simulink model "snap2_f_200msps_64i_4096c_test"  (R2019a)
settings: Solver=VariableStepDiscrete  StartTime=0.0  StopTime=10.0  RelTol=1e-3
libraries: xbsIndex_r4 x8040, casper_library_misc x13, xps_library x6, casper_library_delays x4, casper_library_sources x4, casper_library_reorder x2
(part 11 of 84)

== system snap2_f_200msps_64i_4096c_test/input/bit_stats ==
  din : Inport
  Counter1 : xbsIndex_r4/Counter  cnt_type=Free Running  cnt_to=Inf  operation=Up  start_count=0  cnt_by_val=1  arith_type=Unsigned  n_bits=20  bin_pt=0  load_pin=off  rst=off  en=off  explicit_period=on  period=1  use_behavioral_HDL=off  implementation=Fabric  use_rpm=on  dbl_ovrd=off  block_type=counter
      settings: xl_area=[0, 0, 0, 0, 0, 0, 0]
  Mux : xbsIndex_r4/Mux  inputs=32  en=off  latency=1  precision=Full  arith_type=Unsigned  n_bits=16  bin_pt=14  quantization=Truncate  overflow=Wrap  dbl_ovrd=off  block_type=mux
  Mux1 : xbsIndex_r4/Mux  inputs=2  en=off  latency=1  precision=Full  arith_type=Unsigned  n_bits=16  bin_pt=14  quantization=Truncate  overflow=Wrap  dbl_ovrd=off  block_type=mux
  Slice1 : xbsIndex_r4/Slice  nbits=1  boolean_output=on  mode=Upper Bit Location + Width  bit1=0  base1=MSB of Input  bit0=19  base0=LSB of Input  dbl_ovrd=off  block_type=slice
      settings: infoedit="Extracts a given range of bits from each input sample and presents it at the output.  The output type is ordinarily unsigned with binary point at zero, but can be Boolean when the slice is one bit wide.<P><P>Hardware notes: In hardware this block costs nothing."  block_version=10.1.3
  Slice2 : xbsIndex_r4/Slice  nbits=1  boolean_output=off  mode=Lower Bit Location + Width  bit1=0  base1=MSB of Input  bit0=5  base0=LSB of Input  dbl_ovrd=off  block_type=slice
      settings: block_version=10.1.3
  Slice3 : xbsIndex_r4/Slice  nbits=5  boolean_output=off  mode=Lower Bit Location + Width  bit1=0  base1=MSB of Input  bit0=0  base0=LSB of Input  dbl_ovrd=off  block_type=slice
      settings: block_version=10.1.3
  bus_expand1 : Subsystem  AncestorBlock=casper_library_flow_control/bus_expand  mask(bus_expand){mode=divisions of equal size, outputNum=32, outputWidth=10, outputBinaryPt=0, outputArithmeticType=0, show_format=off, outputToWorkspace=off, variablePrefix=out, outputToModelAsWell=on}
      mask prompts: outputNum "Number of outputs:"; outputWidth "Output width:"; outputBinaryPt "Output binary point position:"; outputArithmeticType "Output arithmetic type (ufix=0, fix=1, bool=2):"; show_format "Print format string?"; outputToWorkspace "Output to workspace?"; variablePrefix "Variable name prefix:"; outputToModelAsWell "Output to model as well?"
      mask help:
      | Expands a 'bus' made using a bus_create or Xilinx
      | concat block.
      | The input will be divided into the specified number
      | of outputs with the specified arithmetic types.
      | Divisions are made from most significant bit.
      mask init: same as snap2_f_200msps_64i_4096c_test/chan_reorder/bus_expand2
      settings: AttributesFormatString=32 outputs
      mask TypeOptions mode: divisions of equal size | divisions of arbitrary size
      mask Callback mode: bus_expand_callback();
      mask Callback outputWidth: bus_expand_callback();
      mask Callback outputToWorkspace: bus_expand_callback();
  bus_expand2 : Subsystem  AncestorBlock=casper_library_flow_control/bus_expand  mask(bus_expand){mode=divisions of equal size, outputNum=2, outputWidth=10*32, outputBinaryPt=0, outputArithmeticType=0, show_format=off, outputToWorkspace=off, variablePrefix=out, outputToModelAsWell=on}
      mask prompts: outputNum "Number of outputs:"; outputWidth "Output width:"; outputBinaryPt "Output binary point position:"; outputArithmeticType "Output arithmetic type (ufix=0, fix=1, bool=2):"; show_format "Print format string?"; outputToWorkspace "Output to workspace?"; variablePrefix "Variable name prefix:"; outputToModelAsWell "Output to model as well?"
      mask help:
      | Expands a 'bus' made using a bus_create or Xilinx
      | concat block.
      | The input will be divided into the specified number
      | of outputs with the specified arithmetic types.
      | Divisions are made from most significant bit.
      mask init: same as snap2_f_200msps_64i_4096c_test/chan_reorder/bus_expand2
      settings: AttributesFormatString=2 outputs
      mask TypeOptions mode: divisions of equal size | divisions of arbitrary size
      mask Callback mode: bus_expand_callback();
      mask Callback outputWidth: bus_expand_callback();
      mask Callback outputToWorkspace: bus_expand_callback();
  edge_detect1 : Subsystem  AncestorBlock=casper_library_misc/edge_detect  mask(edge_detect){edge=Rising, polarity=Active High, x_in=[0 0.08 0.08 0.16 0.16 0.24 0.24 0.32 0.32 0.4], y_in=[-1 -1  1  1  1  1  1  1  1  1], x_out=[0.6 0.68 0.68 0.76 0.76 0.84 0.84 0.92 0.92 1], y_out=[-1 -1  1  1 -1 -1 -1 -1 -1 -1]}
      mask prompts: edge "Edge Type"; polarity "Output Polarity"; x_in "Input X Positions"; y_in "Input Y Positions"; x_out "Output X Positions"; y_out "Output Y Positions"
      mask help: Output is active for one-cycle after each edge of the specified type (i.e. rising, falling or both).
      mask init: same as snap2_f_200msps_64i_4096c_test/sync/ed
      settings: AttributesFormatString=|
      | rising edges
      | active high
      mask Help: Output is active for one-cycle after each edge of the specified type (i.e. rising, falling, or both).  Latency is zero.
      mask TypeOptions edge: Rising | Falling | Both
      mask TypeOptions polarity: Active High | Active Low
      mask Display:
      | plot(x_in_num,0.5+y_in_num*0.2);
      | plot(x_out_num,0.5+y_out_num*0.2);
  histogram : Subsystem  mask{bitwidth=10}
  input_sel : Subsystem  Tag=xps:sw_reg  AncestorBlock=xps_library/Memory/software_register  mask(swreg){io_dir=From Processor, io_delay=0, init_val=0, sample_period=1, names=reg, bitwidths=32, bin_pts=0, arith_types=0, sim_port=on, show_format=on}
      mask prompts: io_dir "I/O direction"; io_delay "I/O delay"; init_val "Initial Value"; sample_period "Sample period"; names "Bitfield names [msb...lsb]"; bitwidths "Bitfield widths"; bin_pts "Bitfield binary pts"; arith_types "Bitfield types, ufix=0, fix=1, bool=2"; sim_port "Provide sim input/output?"; show_format "Print format string?"
      mask help: A 32-bit software-accessible register. Can be divided into bitfields of varying widths and types using the fields in the block mask.
      mask init:
      | swreg_init(gcb)
      settings: AttributesFormatString=1input:uf32.0 = 32 bits
      mask TypeOptions io_dir: To Processor | From Processor
      mask Callback io_dir:
      | mask_enables = get_param(gcb, 'MaskEnables');
      | mask_names = get_param(gcb, 'MaskNames');
      | if strcmp(get_param(gcb, 'io_dir'), 'To Processor'),
      |     mask_enables{ismember(mask_names, 'sample_period')} = 'off';
      | else
      |     mask_enables{ismember(mask_names, 'sample_period')} = 'on';
      | end
      | set_param(gcb, 'MaskEnables', mask_enables);
      mask DialogControl ParameterTabVar0 Prompt: Setup
  wires:
  [adc_hist_rst] -> histogram/2(new_acc)
  Mux/1 -> histogram/1(din)
  Counter1/1 -> Slice1/1
  Slice1/1 -> edge_detect1/1(in)
  edge_detect1/1(out) -> [adc_hist_rst]
  input_sel/1(in_reg) -> Slice3/1, Slice2/1
  Slice2/1 -> [sel_msb]
  din/1 -> bus_expand2/1(bus_in)
  bus_expand2/1(msb_out2) -> Mux1/2
  bus_expand2/2(lsb_out1) -> Mux1/3
  Slice3/1 -> [sel_lsb]
  [sel_msb] -> Mux1/1
  Mux1/1 -> bus_expand1/1(bus_in)
  [sel_lsb] -> Mux/1
  bus_expand1/14(out19) -> Mux/15
  bus_expand1/7(out26) -> Mux/8
  bus_expand1/13(out20) -> Mux/14
  bus_expand1/17(out16) -> Mux/18
  bus_expand1/18(out15) -> Mux/19
  bus_expand1/11(out22) -> Mux/12
  bus_expand1/20(out13) -> Mux/21
  bus_expand1/2(out31) -> Mux/3
  bus_expand1/9(out24) -> Mux/10
  bus_expand1/3(out30) -> Mux/4
  bus_expand1/6(out27) -> Mux/7
  bus_expand1/10(out23) -> Mux/11
  bus_expand1/21(out12) -> Mux/22
  bus_expand1/16(out17) -> Mux/17
  bus_expand1/19(out14) -> Mux/20
  bus_expand1/12(out21) -> Mux/13
  bus_expand1/4(out29) -> Mux/5
  bus_expand1/1(msb_out32) -> Mux/2
  bus_expand1/15(out18) -> Mux/16
  bus_expand1/5(out28) -> Mux/6
  bus_expand1/22(out11) -> Mux/23
  bus_expand1/23(out10) -> Mux/24
  bus_expand1/24(out9) -> Mux/25
  bus_expand1/25(out8) -> Mux/26
  bus_expand1/26(out7) -> Mux/27
  bus_expand1/27(out6) -> Mux/28
  bus_expand1/28(out5) -> Mux/29
  bus_expand1/29(out4) -> Mux/30
  bus_expand1/30(out3) -> Mux/31
  bus_expand1/31(out2) -> Mux/32
  bus_expand1/32(lsb_out1) -> Mux/33
  bus_expand1/8(out25) -> Mux/9

== system snap2_f_200msps_64i_4096c_test/input/bus_create2 ==
  in1 : Inport
  in2 : Inport  Port=2
  in3 : Inport  Port=3
  in4 : Inport  Port=4
  concatenate : xbsIndex_r4/Concat  num_inputs=4  dbl_ovrd=off  block_type=concat
  reinterpret{1..4} (4 alike) : xbsIndex_r4/Reinterpret  force_arith_type=on  arith_type=Unsigned  force_bin_pt=on  bin_pt=0  block_type=reinterpret
      reinterpret1 settings: infoedit="Changes signal type without altering the binary representation.   You can changed the signal between signed and unsigned, and relocate the binary point.<br><br>Hardware notes: In hardware this block costs nothing.<br><br>Example:  Suppose the input is 6 bits wide, signed, with 2 fractional bits, and the output is forced to unsigned with 0 fractional bits.  Then an input of -2.0 (1110.00 in binary 2's complement) becomes an output of 56 (111000 in binary)."
      reinterpret2 settings: infoedit="Changes signal type without altering the binary representation.   You can changed the signal between signed and unsigned, and relocate the binary point.<br><br>Hardware notes: In hardware this block costs nothing.<br><br>Example:  Suppose the input is 6 bits wide, signed, with 2 fractional bits, and the output is forced to unsigned with 0 fractional bits.  Then an input of -2.0 (1110.00 in binary 2's complement) becomes an output of 56 (111000 in binary)."
  bus_out : Outport
  wires:
  concatenate/1 -> bus_out/1
  in1/1 -> reinterpret1/1
  reinterpret1/1 -> concatenate/1
  in2/1 -> reinterpret2/1
  reinterpret2/1 -> concatenate/2
  in3/1 -> reinterpret3/1
  reinterpret3/1 -> concatenate/3
  in4/1 -> reinterpret4/1
  reinterpret4/1 -> concatenate/4

== system snap2_f_200msps_64i_4096c_test/input/bus_mux ==
  sel : Inport
  d0 : Inport  Port=2
  d1 : Inport  Port=3
  d2 : Inport  Port=4
  misci : Inport  Port=5
  d_bussify : Subsystem  AncestorBlock=casper_library_flow_control/bus_create  mask(bus_create){inputNum=64}
      mask prompts: inputNum "Number of inputs:"
      mask init:
      | bus_create_init(gcb,...
      |     'inputNum', inputNum);
  dmisc : xbsIndex_r4/Delay  rst=off  infoeditControl=Selection of Reset will increase slice count due to use of real FFs and instead of SRLs  en=off  latency=1  reg_retiming=on  dbl_ovrd=off  block_type=delay
  expand0 : Subsystem  AncestorBlock=casper_library_flow_control/bus_expand  mask(bus_expand){mode=divisions of arbitrary size, outputNum=1, outputWidth=[10;10;10;10;10;10;10;10;10;10;10;10;10;10;10;10;10;10;10;10;10;10;10;10;10;10;10;10;10;10;10;10;10;10;10;10;10;10;10;10;10;10;10;10;10;10;10;10;10;10;10;10;10;10;10;10;10;10;10;10;10;10;10;10], outputBinaryPt=[0  0  0  0  0  0  0  0  0  0  0  0  0  0  0  0  0  0  0  0  0  0  0  0  0  0  0  0  0  0  0  0  0  0  0  0  0  0  0  0  0  0  0  0  0  0  0  0  0  0  0  0  0  0  0  0  0  0  0  0  0  0  0  0], outputArithmeticType=[0  0  0  0  0  0  0  0  0  0  0  0  0  0  0  0  0  0  0  0  0  0  0  0  0  0  0  0  0  0  0  0  0  0  0  0  0  0  0  0  0  0  0  0  0  0  0  0  0  0  0  0  0  0  0  0  0  0  0  0  0  0  0  0], show_format=on, outputToWorkspace=off, variablePrefix=, outputToModelAsWell=on}
      mask prompts: outputNum "Number of outputs:"; outputWidth "Output width [msb ... lsb]:"; outputBinaryPt "Output binary point position [msb ... lsb]:"; outputArithmeticType "Output arithmetic type (ufix=0, fix=1, bool=2) [msb ... lsb]:"; show_format "Print format string?"; outputToWorkspace "Output to workspace?"; variablePrefix "Variable name prefix:"; outputToModelAsWell "Output to model as well?"
      mask help:
      | Expands a 'bus' made using a bus_create or Xilinx
      | concat block.
      | The input will be divided into the specified number
      | of outputs with the specified arithmetic types.
      | Divisions are made from most significant bit.
      mask init: same as snap2_f_200msps_64i_4096c_test/chan_reorder/bus_expand2
      settings: AttributesFormatString=64 outputs: uf10.0,uf10.0,uf10.0,uf10.0,uf10.0,uf10.0,uf10.0,uf10.0,uf10.0,uf10.0,uf10.0,uf10.0,uf10.0,uf10.0,uf10.0,uf10.0,uf10.0,uf10.0,uf10.0,uf10.0,uf10.0,uf10.0,uf10.0,uf10.0,uf10.0,uf10.0,uf10.0,uf10.0,uf10.0,uf10.0,uf10.0,uf10.0,uf10.0,uf10.0,uf10.0,uf10.0,uf10.0,uf10.0,uf10.0,uf10.0,uf10.0,uf10.0,uf10.0,uf10.0,uf10.0,uf10.0,uf10.0,uf10.0,uf10.0,uf10.0,uf10.0,uf10.0,uf10.0,uf10.0,uf10.0,uf10.0,uf10.0,uf10.0,uf10.0,uf10.0,uf10.0,uf10.0,uf10.0,uf10.0,
      mask TypeOptions mode: divisions of equal size | divisions of arbitrary size
      mask Callback mode: bus_expand_callback();
      mask Callback outputWidth: bus_expand_callback();
      mask Callback outputToWorkspace: bus_expand_callback();
  expand1 : Subsystem  AncestorBlock=casper_library_flow_control/bus_expand  mask(bus_expand){mode=divisions of arbitrary size, outputNum=1, outputWidth=[10;10;10;10;10;10;10;10;10;10;10;10;10;10;10;10;10;10;10;10;10;10;10;10;10;10;10;10;10;10;10;10;10;10;10;10;10;10;10;10;10;10;10;10;10;10;10;10;10;10;10;10;10;10;10;10;10;10;10;10;10;10;10;10], outputBinaryPt=[0  0  0  0  0  0  0  0  0  0  0  0  0  0  0  0  0  0  0  0  0  0  0  0  0  0  0  0  0  0  0  0  0  0  0  0  0  0  0  0  0  0  0  0  0  0  0  0  0  0  0  0  0  0  0  0  0  0  0  0  0  0  0  0], outputArithmeticType=[0  0  0  0  0  0  0  0  0  0  0  0  0  0  0  0  0  0  0  0  0  0  0  0  0  0  0  0  0  0  0  0  0  0  0  0  0  0  0  0  0  0  0  0  0  0  0  0  0  0  0  0  0  0  0  0  0  0  0  0  0  0  0  0], show_format=on, outputToWorkspace=off, variablePrefix=, outputToModelAsWell=on}
      mask prompts: outputNum "Number of outputs:"; outputWidth "Output width [msb ... lsb]:"; outputBinaryPt "Output binary point position [msb ... lsb]:"; outputArithmeticType "Output arithmetic type (ufix=0, fix=1, bool=2) [msb ... lsb]:"; show_format "Print format string?"; outputToWorkspace "Output to workspace?"; variablePrefix "Variable name prefix:"; outputToModelAsWell "Output to model as well?"
      mask help:
      | Expands a 'bus' made using a bus_create or Xilinx
      | concat block.
      | The input will be divided into the specified number
      | of outputs with the specified arithmetic types.
      | Divisions are made from most significant bit.
      mask init: same as snap2_f_200msps_64i_4096c_test/chan_reorder/bus_expand2
      settings: AttributesFormatString=64 outputs: uf10.0,uf10.0,uf10.0,uf10.0,uf10.0,uf10.0,uf10.0,uf10.0,uf10.0,uf10.0,uf10.0,uf10.0,uf10.0,uf10.0,uf10.0,uf10.0,uf10.0,uf10.0,uf10.0,uf10.0,uf10.0,uf10.0,uf10.0,uf10.0,uf10.0,uf10.0,uf10.0,uf10.0,uf10.0,uf10.0,uf10.0,uf10.0,uf10.0,uf10.0,uf10.0,uf10.0,uf10.0,uf10.0,uf10.0,uf10.0,uf10.0,uf10.0,uf10.0,uf10.0,uf10.0,uf10.0,uf10.0,uf10.0,uf10.0,uf10.0,uf10.0,uf10.0,uf10.0,uf10.0,uf10.0,uf10.0,uf10.0,uf10.0,uf10.0,uf10.0,uf10.0,uf10.0,uf10.0,uf10.0,
      mask TypeOptions mode: divisions of equal size | divisions of arbitrary size
      mask Callback mode: bus_expand_callback();
      mask Callback outputWidth: bus_expand_callback();
      mask Callback outputToWorkspace: bus_expand_callback();
  expand2 : Subsystem  AncestorBlock=casper_library_flow_control/bus_expand  mask(bus_expand){mode=divisions of arbitrary size, outputNum=1, outputWidth=[10;10;10;10;10;10;10;10;10;10;10;10;10;10;10;10;10;10;10;10;10;10;10;10;10;10;10;10;10;10;10;10;10;10;10;10;10;10;10;10;10;10;10;10;10;10;10;10;10;10;10;10;10;10;10;10;10;10;10;10;10;10;10;10], outputBinaryPt=[0  0  0  0  0  0  0  0  0  0  0  0  0  0  0  0  0  0  0  0  0  0  0  0  0  0  0  0  0  0  0  0  0  0  0  0  0  0  0  0  0  0  0  0  0  0  0  0  0  0  0  0  0  0  0  0  0  0  0  0  0  0  0  0], outputArithmeticType=[0  0  0  0  0  0  0  0  0  0  0  0  0  0  0  0  0  0  0  0  0  0  0  0  0  0  0  0  0  0  0  0  0  0  0  0  0  0  0  0  0  0  0  0  0  0  0  0  0  0  0  0  0  0  0  0  0  0  0  0  0  0  0  0], show_format=on, outputToWorkspace=off, variablePrefix=, outputToModelAsWell=on}
      mask prompts: outputNum "Number of outputs:"; outputWidth "Output width [msb ... lsb]:"; outputBinaryPt "Output binary point position [msb ... lsb]:"; outputArithmeticType "Output arithmetic type (ufix=0, fix=1, bool=2) [msb ... lsb]:"; show_format "Print format string?"; outputToWorkspace "Output to workspace?"; variablePrefix "Variable name prefix:"; outputToModelAsWell "Output to model as well?"
      mask help:
      | Expands a 'bus' made using a bus_create or Xilinx
      | concat block.
      | The input will be divided into the specified number
      | of outputs with the specified arithmetic types.
      | Divisions are made from most significant bit.
      mask init: same as snap2_f_200msps_64i_4096c_test/chan_reorder/bus_expand2
      settings: AttributesFormatString=64 outputs: uf10.0,uf10.0,uf10.0,uf10.0,uf10.0,uf10.0,uf10.0,uf10.0,uf10.0,uf10.0,uf10.0,uf10.0,uf10.0,uf10.0,uf10.0,uf10.0,uf10.0,uf10.0,uf10.0,uf10.0,uf10.0,uf10.0,uf10.0,uf10.0,uf10.0,uf10.0,uf10.0,uf10.0,uf10.0,uf10.0,uf10.0,uf10.0,uf10.0,uf10.0,uf10.0,uf10.0,uf10.0,uf10.0,uf10.0,uf10.0,uf10.0,uf10.0,uf10.0,uf10.0,uf10.0,uf10.0,uf10.0,uf10.0,uf10.0,uf10.0,uf10.0,uf10.0,uf10.0,uf10.0,uf10.0,uf10.0,uf10.0,uf10.0,uf10.0,uf10.0,uf10.0,uf10.0,uf10.0,uf10.0,
      mask TypeOptions mode: divisions of equal size | divisions of arbitrary size
      mask Callback mode: bus_expand_callback();
      mask Callback outputWidth: bus_expand_callback();
      mask Callback outputToWorkspace: bus_expand_callback();
  mux{0..63} (64 alike) : xbsIndex_r4/Mux  inputs=3  en=off  latency=1  precision=Full  arith_type=Unsigned  n_bits=16  bin_pt=14  quantization=Truncate  overflow=Wrap  dbl_ovrd=off  block_type=mux
  sel_expand : Subsystem  AncestorBlock=casper_library_flow_control/bus_expand  mask(bus_expand){mode=divisions of equal size, outputNum=64, outputWidth=2, outputBinaryPt=0, outputArithmeticType=0, show_format=on, outputToWorkspace=off, variablePrefix=, outputToModelAsWell=on}
      mask prompts: outputNum "Number of outputs:"; outputWidth "Output width:"; outputBinaryPt "Output binary point position:"; outputArithmeticType "Output arithmetic type (ufix=0, fix=1, bool=2):"; show_format "Print format string?"; outputToWorkspace "Output to workspace?"; variablePrefix "Variable name prefix:"; outputToModelAsWell "Output to model as well?"
      mask help:
      | Expands a 'bus' made using a bus_create or Xilinx
      | concat block.
      | The input will be divided into the specified number
      | of outputs with the specified arithmetic types.
      | Divisions are made from most significant bit.
      mask init: same as snap2_f_200msps_64i_4096c_test/chan_reorder/bus_expand2
      settings: AttributesFormatString=64 outputs: uf2.0,uf2.0,uf2.0,uf2.0,uf2.0,uf2.0,uf2.0,uf2.0,uf2.0,uf2.0,uf2.0,uf2.0,uf2.0,uf2.0,uf2.0,uf2.0,uf2.0,uf2.0,uf2.0,uf2.0,uf2.0,uf2.0,uf2.0,uf2.0,uf2.0,uf2.0,uf2.0,uf2.0,uf2.0,uf2.0,uf2.0,uf2.0,uf2.0,uf2.0,uf2.0,uf2.0,uf2.0,uf2.0,uf2.0,uf2.0,uf2.0,uf2.0,uf2.0,uf2.0,uf2.0,uf2.0,uf2.0,uf2.0,uf2.0,uf2.0,uf2.0,uf2.0,uf2.0,uf2.0,uf2.0,uf2.0,uf2.0,uf2.0,uf2.0,uf2.0,uf2.0,uf2.0,uf2.0,uf2.0,
      mask TypeOptions mode: divisions of equal size | divisions of arbitrary size
      mask Callback mode: bus_expand_callback();
      mask Callback outputWidth: bus_expand_callback();
      mask Callback outputToWorkspace: bus_expand_callback();
  out : Outport
  misco : Outport  Port=2
  wires:
  sel/1 -> sel_expand/1(bus_in)
  d0/1 -> expand0/1(bus_in)
  d1/1 -> expand1/1(bus_in)
  d2/1 -> expand2/1(bus_in)
  sel_expand/1(msb_out64) -> mux0/1
  expand0/1(msb_out64) -> mux0/2
  expand1/1(msb_out64) -> mux0/3
  expand2/1(msb_out64) -> mux0/4
  sel_expand/2(out63) -> mux1/1
  expand0/2(out63) -> mux1/2
  expand1/2(out63) -> mux1/3
  expand2/2(out63) -> mux1/4
  sel_expand/3(out62) -> mux2/1
  expand0/3(out62) -> mux2/2
  expand1/3(out62) -> mux2/3
  expand2/3(out62) -> mux2/4
  sel_expand/4(out61) -> mux3/1
  expand0/4(out61) -> mux3/2
  expand1/4(out61) -> mux3/3
  expand2/4(out61) -> mux3/4
  sel_expand/5(out60) -> mux4/1
  expand0/5(out60) -> mux4/2
  expand1/5(out60) -> mux4/3
  expand2/5(out60) -> mux4/4
  sel_expand/6(out59) -> mux5/1
  expand0/6(out59) -> mux5/2
  expand1/6(out59) -> mux5/3
  expand2/6(out59) -> mux5/4
  sel_expand/7(out58) -> mux6/1
  expand0/7(out58) -> mux6/2
  expand1/7(out58) -> mux6/3
  expand2/7(out58) -> mux6/4
  sel_expand/8(out57) -> mux7/1
  expand0/8(out57) -> mux7/2
  expand1/8(out57) -> mux7/3
  expand2/8(out57) -> mux7/4
  sel_expand/9(out56) -> mux8/1
  expand0/9(out56) -> mux8/2
  expand1/9(out56) -> mux8/3
  expand2/9(out56) -> mux8/4
  sel_expand/10(out55) -> mux9/1
  expand0/10(out55) -> mux9/2
  expand1/10(out55) -> mux9/3
  expand2/10(out55) -> mux9/4
  sel_expand/11(out54) -> mux10/1
  expand0/11(out54) -> mux10/2
  expand1/11(out54) -> mux10/3
  expand2/11(out54) -> mux10/4
  sel_expand/12(out53) -> mux11/1
  expand0/12(out53) -> mux11/2
  expand1/12(out53) -> mux11/3
  expand2/12(out53) -> mux11/4
  sel_expand/13(out52) -> mux12/1
  expand0/13(out52) -> mux12/2
  expand1/13(out52) -> mux12/3
  expand2/13(out52) -> mux12/4
  sel_expand/14(out51) -> mux13/1
  expand0/14(out51) -> mux13/2
  expand1/14(out51) -> mux13/3
  expand2/14(out51) -> mux13/4
  sel_expand/15(out50) -> mux14/1
  expand0/15(out50) -> mux14/2
  expand1/15(out50) -> mux14/3
  expand2/15(out50) -> mux14/4
  sel_expand/16(out49) -> mux15/1
  expand0/16(out49) -> mux15/2
  expand1/16(out49) -> mux15/3
  expand2/16(out49) -> mux15/4
  sel_expand/17(out48) -> mux16/1
  expand0/17(out48) -> mux16/2
  expand1/17(out48) -> mux16/3
  expand2/17(out48) -> mux16/4
  sel_expand/18(out47) -> mux17/1
  expand0/18(out47) -> mux17/2
  expand1/18(out47) -> mux17/3
  expand2/18(out47) -> mux17/4
  sel_expand/19(out46) -> mux18/1
  expand0/19(out46) -> mux18/2
  expand1/19(out46) -> mux18/3
  expand2/19(out46) -> mux18/4
  sel_expand/20(out45) -> mux19/1
  expand0/20(out45) -> mux19/2
  expand1/20(out45) -> mux19/3
  expand2/20(out45) -> mux19/4
  sel_expand/21(out44) -> mux20/1
  expand0/21(out44) -> mux20/2
  expand1/21(out44) -> mux20/3
  expand2/21(out44) -> mux20/4
  sel_expand/22(out43) -> mux21/1
  expand0/22(out43) -> mux21/2
  expand1/22(out43) -> mux21/3
  expand2/22(out43) -> mux21/4
  sel_expand/23(out42) -> mux22/1
  expand0/23(out42) -> mux22/2
  expand1/23(out42) -> mux22/3
  expand2/23(out42) -> mux22/4
  sel_expand/24(out41) -> mux23/1
  expand0/24(out41) -> mux23/2
  expand1/24(out41) -> mux23/3
  expand2/24(out41) -> mux23/4
  sel_expand/25(out40) -> mux24/1
  expand0/25(out40) -> mux24/2
  expand1/25(out40) -> mux24/3
  expand2/25(out40) -> mux24/4
  sel_expand/26(out39) -> mux25/1
  expand0/26(out39) -> mux25/2
  expand1/26(out39) -> mux25/3
  expand2/26(out39) -> mux25/4
  sel_expand/27(out38) -> mux26/1
  expand0/27(out38) -> mux26/2
  expand1/27(out38) -> mux26/3
  expand2/27(out38) -> mux26/4
  sel_expand/28(out37) -> mux27/1
  expand0/28(out37) -> mux27/2
  expand1/28(out37) -> mux27/3
  expand2/28(out37) -> mux27/4
  sel_expand/29(out36) -> mux28/1
  expand0/29(out36) -> mux28/2
  expand1/29(out36) -> mux28/3
  expand2/29(out36) -> mux28/4
  sel_expand/30(out35) -> mux29/1
  expand0/30(out35) -> mux29/2
  expand1/30(out35) -> mux29/3
  expand2/30(out35) -> mux29/4
  sel_expand/31(out34) -> mux30/1
  expand0/31(out34) -> mux30/2
  expand1/31(out34) -> mux30/3
  expand2/31(out34) -> mux30/4
  sel_expand/32(out33) -> mux31/1
  expand0/32(out33) -> mux31/2
  expand1/32(out33) -> mux31/3
  expand2/32(out33) -> mux31/4
  sel_expand/33(out32) -> mux32/1
  expand0/33(out32) -> mux32/2
  expand1/33(out32) -> mux32/3
  expand2/33(out32) -> mux32/4
  sel_expand/34(out31) -> mux33/1
  expand0/34(out31) -> mux33/2
  expand1/34(out31) -> mux33/3
  expand2/34(out31) -> mux33/4
  sel_expand/35(out30) -> mux34/1
  expand0/35(out30) -> mux34/2
  expand1/35(out30) -> mux34/3
  expand2/35(out30) -> mux34/4
  sel_expand/36(out29) -> mux35/1
  expand0/36(out29) -> mux35/2
  expand1/36(out29) -> mux35/3
  expand2/36(out29) -> mux35/4
  sel_expand/37(out28) -> mux36/1
  expand0/37(out28) -> mux36/2
  expand1/37(out28) -> mux36/3
  expand2/37(out28) -> mux36/4
  sel_expand/38(out27) -> mux37/1
  expand0/38(out27) -> mux37/2
  expand1/38(out27) -> mux37/3
  expand2/38(out27) -> mux37/4
  sel_expand/39(out26) -> mux38/1
  expand0/39(out26) -> mux38/2
  expand1/39(out26) -> mux38/3
  expand2/39(out26) -> mux38/4
  sel_expand/40(out25) -> mux39/1
  expand0/40(out25) -> mux39/2
  expand1/40(out25) -> mux39/3
  expand2/40(out25) -> mux39/4
  sel_expand/41(out24) -> mux40/1
  expand0/41(out24) -> mux40/2
  expand1/41(out24) -> mux40/3
  expand2/41(out24) -> mux40/4
  sel_expand/42(out23) -> mux41/1
  expand0/42(out23) -> mux41/2
  expand1/42(out23) -> mux41/3
  expand2/42(out23) -> mux41/4
  sel_expand/43(out22) -> mux42/1
  expand0/43(out22) -> mux42/2
  expand1/43(out22) -> mux42/3
  expand2/43(out22) -> mux42/4
  sel_expand/44(out21) -> mux43/1
  expand0/44(out21) -> mux43/2
  expand1/44(out21) -> mux43/3
  expand2/44(out21) -> mux43/4
  sel_expand/45(out20) -> mux44/1
  expand0/45(out20) -> mux44/2
  expand1/45(out20) -> mux44/3
  expand2/45(out20) -> mux44/4
  sel_expand/46(out19) -> mux45/1
  expand0/46(out19) -> mux45/2
  expand1/46(out19) -> mux45/3
  expand2/46(out19) -> mux45/4
  sel_expand/47(out18) -> mux46/1
  expand0/47(out18) -> mux46/2
  expand1/47(out18) -> mux46/3
  expand2/47(out18) -> mux46/4
  sel_expand/48(out17) -> mux47/1
  expand0/48(out17) -> mux47/2
  expand1/48(out17) -> mux47/3
  expand2/48(out17) -> mux47/4
  sel_expand/49(out16) -> mux48/1
  expand0/49(out16) -> mux48/2
  expand1/49(out16) -> mux48/3
  expand2/49(out16) -> mux48/4
  sel_expand/50(out15) -> mux49/1
  expand0/50(out15) -> mux49/2
  expand1/50(out15) -> mux49/3
  expand2/50(out15) -> mux49/4
  sel_expand/51(out14) -> mux50/1
  expand0/51(out14) -> mux50/2
  expand1/51(out14) -> mux50/3
  expand2/51(out14) -> mux50/4
  sel_expand/52(out13) -> mux51/1
  expand0/52(out13) -> mux51/2
  expand1/52(out13) -> mux51/3
  expand2/52(out13) -> mux51/4
  sel_expand/53(out12) -> mux52/1
  expand0/53(out12) -> mux52/2
  expand1/53(out12) -> mux52/3
  expand2/53(out12) -> mux52/4
  sel_expand/54(out11) -> mux53/1
  expand0/54(out11) -> mux53/2
  expand1/54(out11) -> mux53/3
  expand2/54(out11) -> mux53/4
  sel_expand/55(out10) -> mux54/1
  expand0/55(out10) -> mux54/2
  expand1/55(out10) -> mux54/3
  expand2/55(out10) -> mux54/4
  sel_expand/56(out9) -> mux55/1
  expand0/56(out9) -> mux55/2
  expand1/56(out9) -> mux55/3
  expand2/56(out9) -> mux55/4
  sel_expand/57(out8) -> mux56/1
  expand0/57(out8) -> mux56/2
  expand1/57(out8) -> mux56/3
  expand2/57(out8) -> mux56/4
  sel_expand/58(out7) -> mux57/1
  expand0/58(out7) -> mux57/2
  expand1/58(out7) -> mux57/3
  expand2/58(out7) -> mux57/4
  sel_expand/59(out6) -> mux58/1
  expand0/59(out6) -> mux58/2
  expand1/59(out6) -> mux58/3
  expand2/59(out6) -> mux58/4
  sel_expand/60(out5) -> mux59/1
  expand0/60(out5) -> mux59/2
  expand1/60(out5) -> mux59/3
  expand2/60(out5) -> mux59/4
  sel_expand/61(out4) -> mux60/1
  expand0/61(out4) -> mux60/2
  expand1/61(out4) -> mux60/3
  expand2/61(out4) -> mux60/4
  sel_expand/62(out3) -> mux61/1
  expand0/62(out3) -> mux61/2
  expand1/62(out3) -> mux61/3
  expand2/62(out3) -> mux61/4
  sel_expand/63(out2) -> mux62/1
  expand0/63(out2) -> mux62/2
  expand1/63(out2) -> mux62/3
  expand2/63(out2) -> mux62/4
  sel_expand/64(lsb_out1) -> mux63/1
  expand0/64(lsb_out1) -> mux63/2
  expand1/64(lsb_out1) -> mux63/3
  expand2/64(lsb_out1) -> mux63/4
  misci/1 -> dmisc/1
  mux0/1 -> d_bussify/1(in1)
  mux1/1 -> d_bussify/2(in2)
  mux2/1 -> d_bussify/3(in3)
  mux3/1 -> d_bussify/4(in4)
  mux4/1 -> d_bussify/5(in5)
  mux5/1 -> d_bussify/6(in6)
  mux6/1 -> d_bussify/7(in7)
  mux7/1 -> d_bussify/8(in8)
  mux8/1 -> d_bussify/9(in9)
  mux9/1 -> d_bussify/10(in10)
  mux10/1 -> d_bussify/11(in11)
  mux11/1 -> d_bussify/12(in12)
  mux12/1 -> d_bussify/13(in13)
  mux13/1 -> d_bussify/14(in14)
  mux14/1 -> d_bussify/15(in15)
  mux15/1 -> d_bussify/16(in16)
  mux16/1 -> d_bussify/17(in17)
  mux17/1 -> d_bussify/18(in18)
  mux18/1 -> d_bussify/19(in19)
  mux19/1 -> d_bussify/20(in20)
  mux20/1 -> d_bussify/21(in21)
  mux21/1 -> d_bussify/22(in22)
  mux22/1 -> d_bussify/23(in23)
  mux23/1 -> d_bussify/24(in24)
  mux24/1 -> d_bussify/25(in25)
  mux25/1 -> d_bussify/26(in26)
  mux26/1 -> d_bussify/27(in27)
  mux27/1 -> d_bussify/28(in28)
  mux28/1 -> d_bussify/29(in29)
  mux29/1 -> d_bussify/30(in30)
  mux30/1 -> d_bussify/31(in31)
  mux31/1 -> d_bussify/32(in32)
  mux32/1 -> d_bussify/33(in33)
  mux33/1 -> d_bussify/34(in34)
  mux34/1 -> d_bussify/35(in35)
  mux35/1 -> d_bussify/36(in36)
  mux36/1 -> d_bussify/37(in37)
  mux37/1 -> d_bussify/38(in38)
  mux38/1 -> d_bussify/39(in39)
  mux39/1 -> d_bussify/40(in40)
  mux40/1 -> d_bussify/41(in41)
  mux41/1 -> d_bussify/42(in42)
  mux42/1 -> d_bussify/43(in43)
  mux43/1 -> d_bussify/44(in44)
  mux44/1 -> d_bussify/45(in45)
  mux45/1 -> d_bussify/46(in46)
  mux46/1 -> d_bussify/47(in47)
  mux47/1 -> d_bussify/48(in48)
  mux48/1 -> d_bussify/49(in49)
  mux49/1 -> d_bussify/50(in50)
  mux50/1 -> d_bussify/51(in51)
  mux51/1 -> d_bussify/52(in52)
  mux52/1 -> d_bussify/53(in53)
  mux53/1 -> d_bussify/54(in54)
  mux54/1 -> d_bussify/55(in55)
  mux55/1 -> d_bussify/56(in56)
  mux56/1 -> d_bussify/57(in57)
  mux57/1 -> d_bussify/58(in58)
  mux58/1 -> d_bussify/59(in59)
  mux59/1 -> d_bussify/60(in60)
  mux60/1 -> d_bussify/61(in61)
  mux61/1 -> d_bussify/62(in62)
  mux62/1 -> d_bussify/63(in63)
  mux63/1 -> d_bussify/64(in64)
  d_bussify/1(bus_out) -> out/1
  dmisc/1 -> misco/1

== system snap2_f_200msps_64i_4096c_test/input/chan_slice ==
  sel : Inport
  din : Inport  Port=2
  sync_in : Inport  Port=3
  Delay : xbsIndex_r4/Delay  rst=off  infoeditControl=Selection of Reset will increase slice count due to use of real FFs and instead of SRLs  en=off  latency=1  reg_retiming=on  dbl_ovrd=off  block_type=delay
  Delay1 : xbsIndex_r4/Delay  rst=off  infoeditControl=Selection of Reset will increase slice count due to use of real FFs and instead of SRLs  en=off  latency=1  reg_retiming=on  dbl_ovrd=off  block_type=delay
  Mux : xbsIndex_r4/Mux  inputs=8  en=off  latency=1  precision=Full  arith_type=Unsigned  n_bits=16  bin_pt=14  quantization=Truncate  overflow=Wrap  dbl_ovrd=off  block_type=mux
  Mux1 : xbsIndex_r4/Mux  inputs=8  en=off  latency=1  precision=Full  arith_type=Unsigned  n_bits=16  bin_pt=14  quantization=Truncate  overflow=Wrap  dbl_ovrd=off  block_type=mux
  bus_expand : Subsystem  AncestorBlock=casper_library_flow_control/bus_expand  mask(bus_expand){mode=divisions of equal size, outputNum=8, outputWidth=10*8, outputBinaryPt=0, outputArithmeticType=0, show_format=off, outputToWorkspace=off, variablePrefix=out, outputToModelAsWell=on}
      mask prompts: outputNum "Number of outputs:"; outputWidth "Output width:"; outputBinaryPt "Output binary point position:"; outputArithmeticType "Output arithmetic type (ufix=0, fix=1, bool=2):"; show_format "Print format string?"; outputToWorkspace "Output to workspace?"; variablePrefix "Variable name prefix:"; outputToModelAsWell "Output to model as well?"
      mask help:
      | Expands a 'bus' made using a bus_create or Xilinx
      | concat block.
      | The input will be divided into the specified number
      | of outputs with the specified arithmetic types.
      | Divisions are made from most significant bit.
      mask init: same as snap2_f_200msps_64i_4096c_test/chan_reorder/bus_expand2
      settings: AttributesFormatString=8 outputs
      mask TypeOptions mode: divisions of equal size | divisions of arbitrary size
      mask Callback mode: bus_expand_callback();
      mask Callback outputWidth: bus_expand_callback();
      mask Callback outputToWorkspace: bus_expand_callback();
  bus_expand1 : Subsystem  AncestorBlock=casper_library_flow_control/bus_expand  mask(bus_expand){mode=divisions of equal size, outputNum=8, outputWidth=10, outputBinaryPt=0, outputArithmeticType=0, show_format=off, outputToWorkspace=off, variablePrefix=out, outputToModelAsWell=on}
      mask prompts: outputNum "Number of outputs:"; outputWidth "Output width:"; outputBinaryPt "Output binary point position:"; outputArithmeticType "Output arithmetic type (ufix=0, fix=1, bool=2):"; show_format "Print format string?"; outputToWorkspace "Output to workspace?"; variablePrefix "Variable name prefix:"; outputToModelAsWell "Output to model as well?"
      mask help:
      | Expands a 'bus' made using a bus_create or Xilinx
      | concat block.
      | The input will be divided into the specified number
      | of outputs with the specified arithmetic types.
      | Divisions are made from most significant bit.
      mask init: same as snap2_f_200msps_64i_4096c_test/chan_reorder/bus_expand2
      settings: AttributesFormatString=8 outputs
      mask TypeOptions mode: divisions of equal size | divisions of arbitrary size
      mask Callback mode: bus_expand_callback();
      mask Callback outputWidth: bus_expand_callback();
      mask Callback outputToWorkspace: bus_expand_callback();
  slice1 : xbsIndex_r4/Slice  nbits=3  boolean_output=off  mode=Lower Bit Location + Width  bit1=0  base1=MSB of Input  bit0=0  base0=LSB of Input  dbl_ovrd=off  block_type=slice
  slice2 : xbsIndex_r4/Slice  nbits=3  boolean_output=off  mode=Lower Bit Location + Width  bit1=0  base1=MSB of Input  bit0=3  base0=LSB of Input  dbl_ovrd=off  block_type=slice
  dout : Outport
  sync_out : Outport  Port=2
  wires:
  bus_expand/2(out7) -> Mux1/3
  Mux1/1 -> bus_expand1/1(bus_in)
  bus_expand/4(out5) -> Mux1/5
  bus_expand1/2(out7) -> Mux/3
  bus_expand1/3(out6) -> Mux/4
  bus_expand/3(out6) -> Mux1/4
  bus_expand1/7(out2) -> Mux/8
  bus_expand1/6(out3) -> Mux/7
  Delay1/1 -> sync_out/1
  sync_in/1 -> Delay/1
  bus_expand/6(out3) -> Mux1/7
  sel/1 -> slice2/1, slice1/1
  bus_expand/1(msb_out8) -> Mux1/2
  din/1 -> bus_expand/1(bus_in)
  bus_expand1/8(lsb_out1) -> Mux/9
  Mux/1 -> dout/1
  bus_expand1/4(out5) -> Mux/5
  slice1/1 -> Mux/1
  bus_expand/5(out4) -> Mux1/6
  Delay/1 -> Delay1/1
  bus_expand1/5(out4) -> Mux/6
  bus_expand1/1(msb_out8) -> Mux/2
  slice2/1 -> Mux1/1
  bus_expand/7(out2) -> Mux1/8
  bus_expand/8(lsb_out1) -> Mux1/9
